simulink model "Mass_Spring_System"  (R2014a)
settings: Solver=ode45  StartTime=0.0  StopTime=StopTime  FixedStep=0.01  MaxStep=0.01  RelTol=1e-3
values from neighbouring files (symbols this model uses):
  b = 10    [Mass_Spring_Damper_System.m]
  F = 0    [Mass_Spring_Damper_System.m]
  K = 400    [Mass_Spring_Damper_System.m]
  m = massValues(i)    [Mass_Spring_Damper_System.m]
  x0 = 1    [Mass_Spring_Damper_System.m]
settings Model: Creator=Omar Emad  LastModifiedBy=Omar Emad
settings DataIOCC: MaxDataPoints=2000  SaveCompleteFinalSimState=on  SaveOutput=off  SaveTime=off  OutputTimes=10
settings DebuggingCC: SolverPrmCheckMsg=none

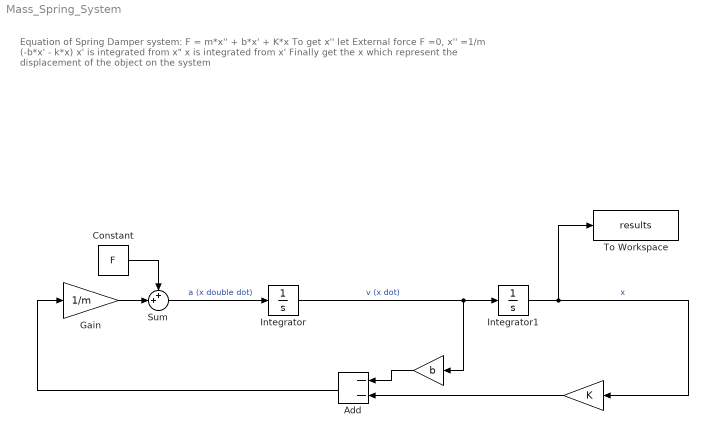
== system Mass_Spring_System ==
  note: Equation of Spring Damper system:
      |
      | F = m*x'' + b*x' + K*x
      | To get x'' let External force F =0, x'' =1/m (-b*x' - k*x)
      | x' is integrated from x"
      | x is integrated from x'
      |
      | Finally get the x which represent the displacement of the object on the system
  " " : Gain  Gain=b
  "  " : Gain  Gain=K
  Add : Sum  Inputs=--
  Constant : Constant  Value=F
  Gain : Gain  Gain=1/m
  Integrator : Integrator
  Integrator1 : Integrator  InitialCondition=x0
  Sum : Sum  Inputs=++|
  To Workspace : ToWorkspace  VariableName=results  SaveFormat=Timeseries  SampleTime=-1
  wires:
  Add/1 -> Gain/1
  Integrator/1 -> " "/1, Integrator1/1  "v (x dot)"
  Integrator1/1 -> To Workspace/1, "  "/1  "x"
  " "/1 -> Add/1
  "  "/1 -> Add/2
  Gain/1 -> Sum/2
  Sum/1 -> Integrator/1  "a (x double dot)"
  Constant/1 -> Sum/1
